simulink model "Utilizando_BUS"  (R2013b)
settings: Solver=ode45  StartTime=0.0  StopTime=10.0  RelTol=1e-3
InitFcn:
  | load('bus_structure.mat');
settings Model: Creator=Eduardo  LastModifiedBy=Eduardo

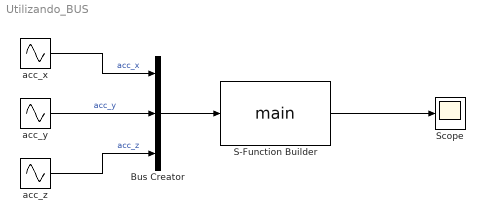
== system Utilizando_BUS ==
  Bus Creator : BusCreator  Inputs=3  OutDataTypeStr=Bus: Aceleracao
  S-Function Builder : S-Function  InitFcn=try, set_param(gcb,'FunctionName','main'), end  FunctionName=main  SFunctionModules=main_wrapper agua  EnableBusSupport=off  mask(S-Function Builder){}
      mask help: Simulink:masks:SFunctionBuilder_MD
      mask init:
      | val = [[.9  0.75 0.75 1 1 .9 .9 1]',[1 1 0.75 0.75 .9 .9 1 .9]'];try , sys = get_param(gcb,'SfunBuilderFcnName');if isempty(sys), sys = get_param(gcb,'FunctionName'); end,catch, sys = get_param(gcb,'FunctionName'); end
      settings: CopyFcn=set_param(gcbh,'LinkStatus','none')  PreSaveFcn=try, set_param(gcb,'FunctionName','main'), end  OpenFcn=sfunctionwizard(gcbh)
      mask Display:
      | plot(val(:,1),val(:,2))
      | disp(sys)
      | port_label('input',1,'In')
      | port_label('output',1,'Out')
  Scope : Scope
  acc_x : Sin  Phase=0.5  SampleTime=0
  acc_y : Sin  Phase=0.5  SampleTime=0
  acc_z : Sin  Phase=1  SampleTime=0
  wires:
  acc_x/1 -> Bus Creator/1  "acc_x"
  acc_y/1 -> Bus Creator/2  "acc_y"
  acc_z/1 -> Bus Creator/3  "acc_z"
  Bus Creator/1 -> S-Function Builder/1
  S-Function Builder/1 -> Scope/1
